simulink model "FI_tpl"  (R2017b)
settings: Solver=VariableStepAuto  StartTime=0  StopTime=254.93  FixedStep=dt_sim  MaxStep=0.1  RelTol=1e-6  EnableMultiTasking=on
values from neighbouring files (symbols this model uses):
  Amp = PARGRID(1,icase)    [run_FI.m]
  corr_select = zeros(1,ny)    [run_FI.m]
  DC = [PARGRID(2,icase) PARGRID(3,icase)]    [run_FI.m]
  t0 = 2    [run_FI.m]
  tstart = T(1)    [LissajouFig.m]    (also in run_FI.m = t0+ncyc(irun)/w_Hz+10)
  w = frq(irun)    [run_FI.m]
  w_Hz = w/2/pi    (= 0.0159154943092)    [run_FI.m]
undefined symbols (not defined in the file or in its folder): AAF_DEN, AAF_NUM, DiscIntNeverNeededParam, dt_sim
libraries: cstblocks x1, dspstat3 x1
settings Model: SimulationMode=accelerator  Creator=Alon  LastModifiedBy=RubinDan
settings DataIOCC: SaveFormat=Array  SignalLoggingSaveFormat=ModelDataLogs  SaveOutput=off  SignalLogging=off  DSMLogging=off  SaveTime=off
settings OptimizationCC: ExpressionDepthLimit=2147483647  EfficientMapNaN2IntZero=off  LifeSpan=inf
settings DebuggingCC: UnderspecifiedInitializationDetection=Classic  MergeDetectMultiDrivingBlocksExec=none  SolverPrmCheckMsg=warning  FcnCallInpInsideContextMsg=warning  StateNameClashWarn=warning  SFUnexpectedBacktrackingDiag=warning  SFNoUnconditionalDefaultTransitionDiag=warning  SFExecutionAtInitializationDiag=none
settings HardwareCC: ProdBitPerPointer=32  ProdBitPerSizeT=32  ProdBitPerPtrDiffT=32  ProdLargestAtomicFloat=None  ProdIntDivRoundTo=Undefined  ProdEndianess=Unspecified  ProdWordSize=32  ProdHWDeviceType=32-bit Generic  TargetBitPerPointer=64  TargetBitPerSizeT=64  TargetBitPerPtrDiffT=64  TargetLongLongMode=on  TargetIntDivRoundTo=Zero  TargetEndianess=LittleEndian  TargetWordSize=64  TargetHWDeviceType=MATLAB Host  ProdEqTarget=off
settings ModelReferenceCC: PropagateSignalLabelsOutOfModel=off
settings SFSimCC: SimParseCustomCode=off
settings CodeAppCC: MaxIdLength=128  StateflowObjectComments=on
settings GRTTargetCC: TargetLangStandard=C89/C90 (ANSI)  CombineOutputUpdateFcns=off  GRTInterface=on
settings ConfigComp: CovMetricSettings=dw  CovHtmlReporting=on  CovSaveCumulativeToWorkspaceVar=on  CovSaveSingleToWorkspaceVar=on  CovExternalEMLEnable=off  CovSFcnEnable=off
settings SimscapeCC: EditingMode=Restricted

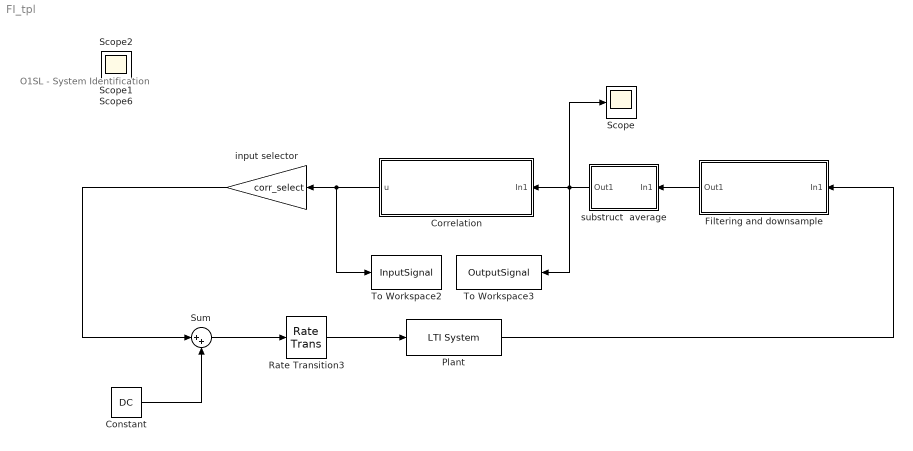
== system FI_tpl ==
  note: O1SL - System Identification
  Constant : Constant  Value=DC  SampleTime=dt_sim
  Correlation : Subsystem
  Filtering and downsample : Subsystem
  Plant : cstblocks/LTI System  sys=P  IC=[]
  Rate Transition3 : RateTransition  OutPortSampleTime=0
  Scope{,1..2,6} (4 alike) : Scope
  Sum : Sum  Inputs=|++
  To Workspace2 : ToWorkspace  VariableName=InputSignal  SaveFormat=Structure With Time  SampleTime=-1
      settings: MaxDataPoints=Np
  To Workspace3 : ToWorkspace  VariableName=OutputSignal  SaveFormat=Structure With Time  SampleTime=-1
      settings: MaxDataPoints=Np
  input selector : Gain  Gain=corr_select
  substruct  average : Subsystem  mask{T_start=tstart, T_sample=dt_sim}
      mask prompts: T_start "Start Time"; T_sample "Smaple Time"
  wires:
  Plant/1 -> Filtering and downsample/1(In1)
  Filtering and downsample/1(Out1) -> substruct  average/1(In1)
  Sum/1 -> Rate Transition3/1
  Constant/1 -> Sum/2
  input selector/1 -> Sum/1
  Rate Transition3/1 -> Plant/1
  substruct  average/1(Out1) -> Scope/1, To Workspace3/1, Correlation/1(In1)
  Correlation/1(u) -> To Workspace2/1, input selector/1

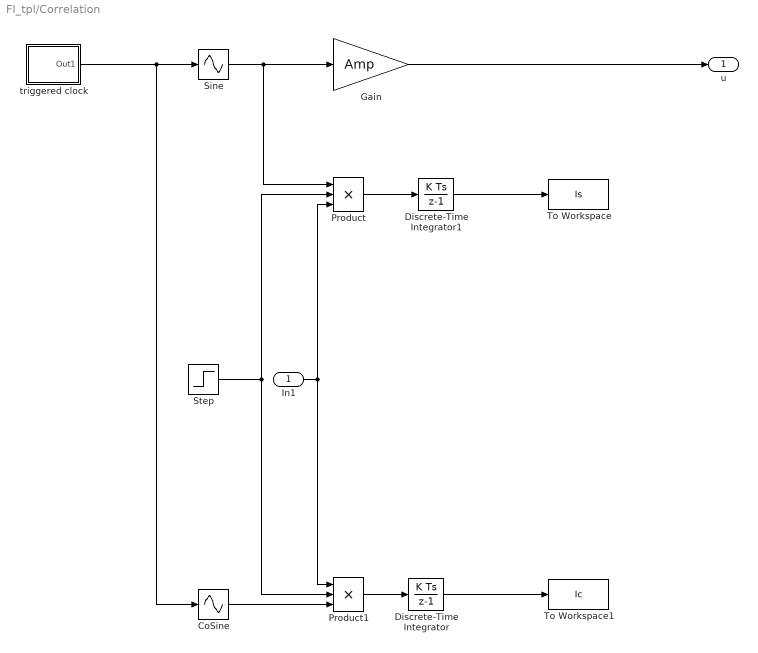
== system FI_tpl/Correlation ==
  In1 : Inport
  CoSine : Sin  TimeSource=Use external signal  Frequency=w  Phase=pi/2  SampleTime=0.001
  Discrete-Time Integrator : DiscreteIntegrator  SampleTime=dt_sim  ICPrevOutput=DiscIntNeverNeededParam  ICPrevScaledInput=DiscIntNeverNeededParam
  Discrete-Time Integrator1 : DiscreteIntegrator  SampleTime=dt_sim  ICPrevOutput=DiscIntNeverNeededParam  ICPrevScaledInput=DiscIntNeverNeededParam
  Gain : Gain  Gain=Amp
  Product : Product  Inputs=3  RndMeth=Zero
  Product1 : Product  Inputs=3  RndMeth=Zero
  Sine : Sin  TimeSource=Use external signal  Frequency=w  SampleTime=0.001
  Step : Step  Time=tstart  SampleTime=dt_sim
  To Workspace : ToWorkspace  VariableName=Is  SaveFormat=Structure  SampleTime=-1
  To Workspace1 : ToWorkspace  VariableName=Ic  SaveFormat=Structure  SampleTime=-1
  triggered clock : Subsystem  mask{T_start=t0, T_sample=dt_sim}
      mask prompts: T_start "Start Time"; T_sample "Smaple Time"
  u : Outport
  wires:
  Sine/1 -> Product/1, Gain/1
  triggered clock/1(Out1) -> CoSine/1, Sine/1
  Product/1 -> Discrete-Time Integrator1/1
  Product1/1 -> Discrete-Time Integrator/1
  Discrete-Time Integrator1/1 -> To Workspace/1
  Discrete-Time Integrator/1 -> To Workspace1/1
  Gain/1 -> u/1
  In1/1 -> Product1/1, Product/3
  Step/1 -> Product1/2, Product/2
  CoSine/1 -> Product1/3

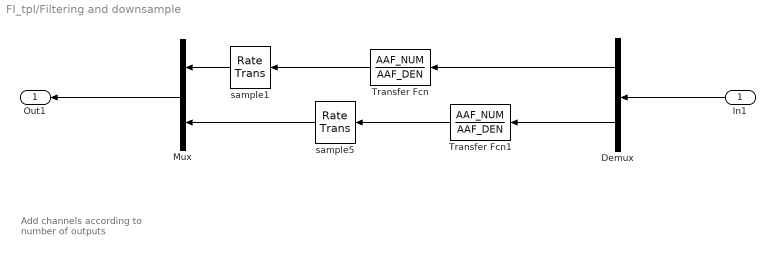
== system FI_tpl/Filtering and downsample ==
  note: Add channels according to number of outputs
  In1 : Inport
  Demux : Demux  Outputs=2
  Mux : Mux  Inputs=2
  Transfer Fcn : TransferFcn  Numerator=AAF_NUM  Denominator=AAF_DEN
  Transfer Fcn1 : TransferFcn  Numerator=AAF_NUM  Denominator=AAF_DEN
  sample1 : RateTransition  OutPortSampleTime=dt_sim
  sample5 : RateTransition  OutPortSampleTime=dt_sim
  Out1 : Outport
  wires:
  Demux/2 -> Transfer Fcn1/1
  Demux/1 -> Transfer Fcn/1
  Mux/1 -> Out1/1
  Transfer Fcn/1 -> sample1/1
  Transfer Fcn1/1 -> sample5/1
  sample5/1 -> Mux/2
  sample1/1 -> Mux/1
  In1/1 -> Demux/1

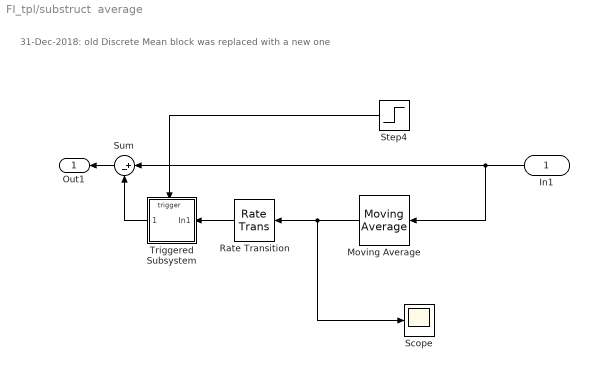
== system FI_tpl/substruct  average ==
  note: 31-Dec-2018: old Discrete Mean block was replaced with a new one
  In1 : Inport
  Moving Average : dspstat3/Moving Average  Method=Sliding window  SpecifyWindowLength=on  WindowLength=2*ceil(1/w_Hz/dt_sim)  ForgettingFactor=0.9  SimulateUsing=Code generation
  Rate Transition : RateTransition
  Scope : Scope
  Step4 : Step  Time=T_start  SampleTime=T_sample
  Sum : Sum  Inputs=|+-
  Triggered Subsystem : Subsystem  TreatAsAtomicUnit=on
  Out1 : Outport
  wires:
  Sum/1 -> Out1/1
  Triggered Subsystem/1(Out1) -> Sum/2
  Step4/1 -> Triggered Subsystem/Trigger
  In1/1 -> Moving Average/1, Sum/1
  Moving Average/1 -> Scope/1, Rate Transition/1
  Rate Transition/1 -> Triggered Subsystem/1(In1)

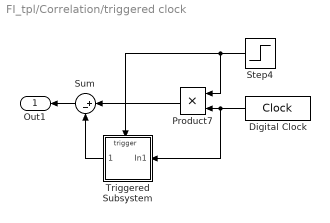
== system FI_tpl/Correlation/triggered clock ==
  Digital Clock : DigitalClock  SampleTime=T_sample
  Product7 : Product  RndMeth=Zero
  Step4 : Step  Time=T_start  SampleTime=T_sample
  Sum : Sum  Inputs=|+-
  Triggered Subsystem : Subsystem  TreatAsAtomicUnit=on
  Out1 : Outport
  wires:
  Step4/1 -> Triggered Subsystem/Trigger, Product7/1
  Digital Clock/1 -> Product7/2, Triggered Subsystem/1(In1)
  Product7/1 -> Sum/1
  Triggered Subsystem/1(Out1) -> Sum/2
  Sum/1 -> Out1/1

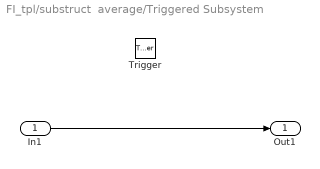
== system FI_tpl/substruct  average/Triggered Subsystem ==
  In1 : Inport
  Trigger : TriggerPort  VariantControl=Variant
  Out1 : Outport
  wires:
  In1/1 -> Out1/1

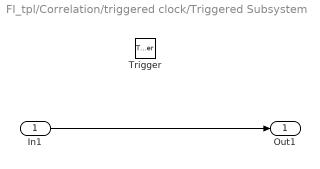
== system FI_tpl/Correlation/triggered clock/Triggered Subsystem ==
  In1 : Inport
  Trigger : TriggerPort  VariantControl=Variant
  Out1 : Outport
  wires:
  In1/1 -> Out1/1
